simulink model "Exercise21"  (R2017a)
settings: Solver=VariableStepAuto  StartTime=0.0  StopTime=10.0  MaxStep=0.002  RelTol=1e-3
undefined symbols (not defined in the file): Freq
settings Model: Creator=JakobLab  LastModifiedBy=JakobLab

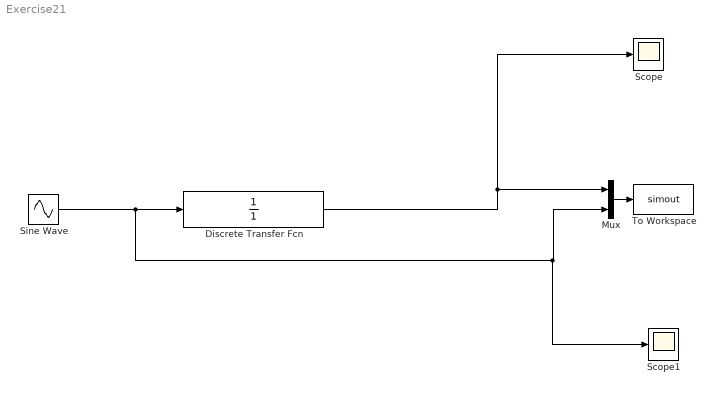
== system Exercise21 ==
  Discrete Transfer Fcn : DiscreteTransferFcn  Denominator=[1]  SampleTime=0.1
  Mux : Mux  Inputs=2
  Scope : Scope
  Scope1 : Scope
  Sine Wave : Sin  Frequency=Freq  SampleTime=0
  To Workspace : ToWorkspace  VariableName=simout  SaveFormat=Structure With Time  SampleTime=-1
  wires:
  Discrete Transfer Fcn/1 -> Mux/1, Scope/1
  Sine Wave/1 -> Scope1/1, Mux/2, Discrete Transfer Fcn/1
  Mux/1 -> To Workspace/1
